simulink model "to_point"  (R2023b)
settings: Solver=FixedStepAuto  StartTime=0.0  StopTime=inf  RelTol=1e-3  EnableMultiTasking=on
model workspace (MAT data in the model file):
  G = 2001
undefined symbols (not defined in the file): c_t, f_max, f_min, Kd, Kp, M, W
libraries: rpi_blkst x2, robotcorelib x1
settings Model: ExtModeTrigDuration=2  Creator=yabde  LastModifiedBy=yabde
settings SolverCC: PositivePriorityOrder=on
settings OptimizationCC: EnhancedBackFolding=on  PassReuseOutputArgsAs=Individual arguments  ZeroExternalMemoryAtStartup=off  ZeroInternalMemoryAtStartup=off  MaxStackSize=64  OptimizeBlockOrder=speed  DifferentSizesBufferReuse=on  OptimizationCustomize=off  EfficientTunableParamExpr=on
settings DebuggingCC: ParameterTunabilityLossMsg=error
settings HardwareCC: ProdBitPerLong=64  ProdLargestAtomicInteger=LongLong  ProdLargestAtomicFloat=Double  ProdLongLongMode=on  ProdHWDeviceType=ARM Compatible->ARM 64-bit (LP64)
settings RTWCC: Description=Embedded Coder  SystemTargetFile=ert.tlc  HardwareBoard=Raspberry Pi (64bit)  TLCOptions="-aInlineSetEventsForThisBaseRateFcn=TLC_FALSE -aSuppressMultiTaskScheduler=TLC_FALSE  -aRateBasedStepFcn=0"  TemplateMakefile=ert_default_tmf  Toolchain=GNU GCC Embedded Linux  BuildConfiguration=Faster Runs
settings CodeAppCC: ForceParamTrailComments=on  IgnoreCustomStorageClasses=off  OperatorAnnotations=on  SimulinkDataObjDesc=on  SFDataObjDesc=on  InsertBlockDesc=on
settings ERTTargetCC: SupportVariableSizeSignals=on  ExtModeTransport=2  ExtModeStaticAlloc=on  ExtModeMexFile=ext_xcp  ExtModeIntrfLevel=Level2 - Open

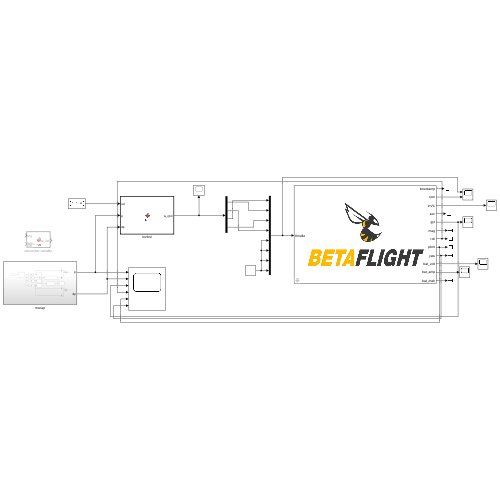
[thumbnail: Simulink's stored preview of the top-level diagram]
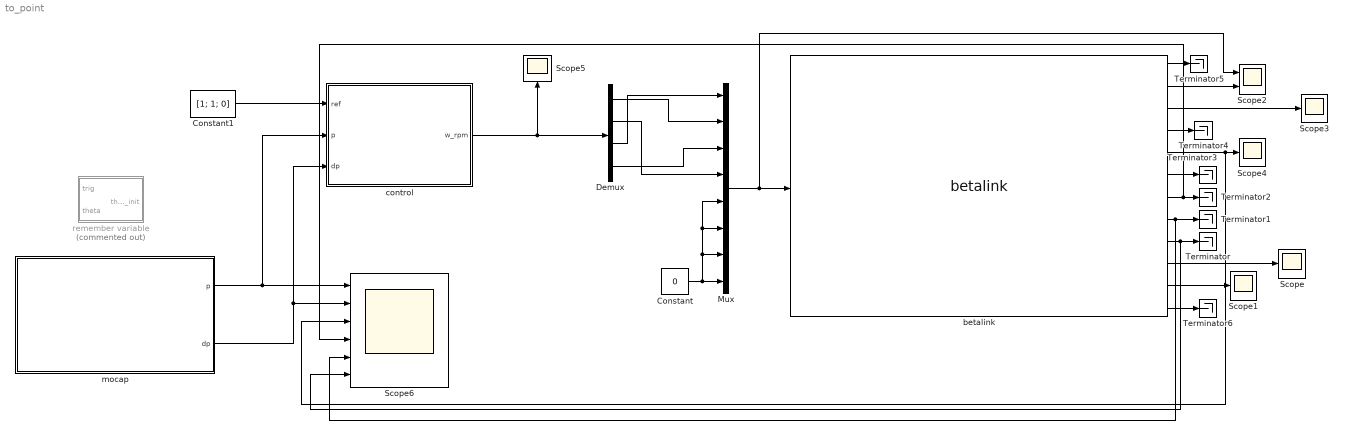
== system to_point ==
  Constant : Constant  Value=0
  Constant1 : Constant  Value=[1; 1; 0]
  Demux : Demux
  Mux : Mux  Inputs=8
  Scope{,1,3..5} (5 alike) : Scope
  Scope2 : Scope  NumInputPorts=2
  Scope6 : Scope  NumInputPorts=6
  Terminator{,1..6} (7 alike) : Terminator
  betalink : rpi_blkst/betalink  rpi_mask_usb_serial_number=1042260556  rpi_mask_Ts=0.01
      settings: SourceProductName=RPI Blockset
  control : MATLAB Function  TreatAsAtomicUnit=on
  mocap : Subsystem
  remember variable : MATLAB Function  Commented=on  TreatAsAtomicUnit=on
  wires:
  Mux/1 -> betalink/1, Scope2/1
  Constant/1 -> Mux/5, Mux/6, Mux/7, Mux/8
  betalink/10 -> Scope/1
  betalink/11 -> Scope1/1
  betalink/2 -> Scope2/2
  betalink/3 -> Scope3/1
  betalink/5 -> Scope6/3, Scope4/1
  betalink/9 -> Scope6/6, Terminator/1
  betalink/8 -> Scope6/5, Terminator1/1
  betalink/7 -> Scope6/4, Terminator2/1
  betalink/6 -> Terminator3/1
  betalink/4 -> Terminator4/1
  betalink/12 -> Terminator6/1
  betalink/1 -> Terminator5/1
  mocap/2(dp) -> control/3(dp), Scope6/2
  control/1(w_rpm) -> Demux/1, Scope5/1
  Demux/1 -> Mux/2
  Demux/2 -> Mux/4
  Demux/3 -> Mux/1
  Demux/4 -> Mux/3
  mocap/1(p) -> control/2(p), Scope6/1
  Constant1/1 -> control/1(ref)

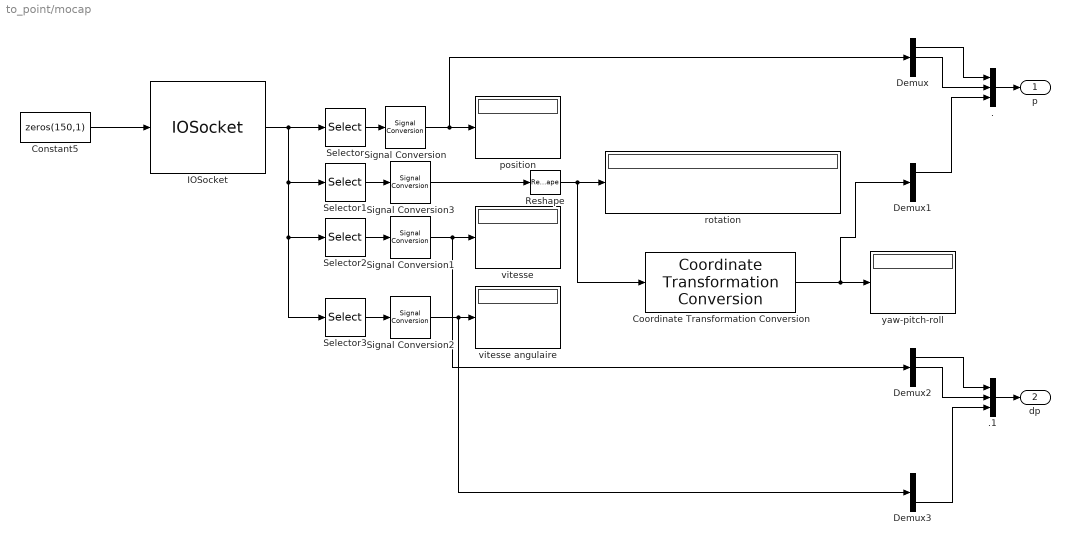
== system to_point/mocap ==
  . : Mux  Inputs=3
  .1 : Mux  Inputs=3
  Constant5 : Constant  Value=zeros(150,1)
  Coordinate Transformation Conversion : robotcorelib/Coordinate Transformation Conversion  InputRepresentation=Rotation Matrix  InputEulerSequence=ZYX  ShowTrVecInputPort=on  OutputRepresentation=Euler Angles  OutputEulerSequence=ZYX  ShowTrVecOutputPort=on  SimulateUsing=Interpreted execution
  Demux{,1..3} (4 alike) : Demux  Outputs=3
  IOSocket : rpi_blkst/IOSocket  rpi_mask_Ts=0.01  rpi_mask_ip1=192  rpi_mask_ip2=168  rpi_mask_ip3=0  rpi_mask_ip4=13  rpi_mask_port=31415
      settings: SourceProductName=RPI Blockset
  Reshape : Reshape  OutputDimensionality=Customize  OutputDimensions=[3,3]
  Selector : Selector  IndexOptions=Index vector (dialog)  Indices=3:5  OutputSizes=1
  Selector1 : Selector  IndexOptions=Index vector (dialog)  Indices=6:14  OutputSizes=1
  Selector2 : Selector  IndexOptions=Index vector (dialog)  Indices=15:17  OutputSizes=1
  Selector3 : Selector  IndexOptions=Index vector (dialog)  Indices=18:20  OutputSizes=1
  Signal Conversion{,1..3} (4 alike) : SignalConversion  OverrideOpt=off
  position : Display
  rotation : Display
  vitesse : Display
  vitesse angulaire : Display
  yaw-pitch-roll : Display
  p : Outport
  dp : Outport  Port=2
  wires:
  Selector2/1 -> Signal Conversion1/1
  Signal Conversion1/1 -> Demux2/1, vitesse/1
  Signal Conversion2/1 -> Demux3/1, vitesse angulaire/1
  Selector/1 -> Signal Conversion/1
  Constant5/1 -> IOSocket/1
  Reshape/1 -> Coordinate Transformation Conversion/1, rotation/1
  IOSocket/1 -> Selector3/1, Selector2/1, Selector1/1, Selector/1
  Selector3/1 -> Signal Conversion2/1
  Signal Conversion/1 -> Demux/1, position/1
  Selector1/1 -> Signal Conversion3/1
  Signal Conversion3/1 -> Reshape/1
  Coordinate Transformation Conversion/1 -> Demux1/1, yaw-pitch-roll/1
  Demux/1 -> ./1
  Demux/2 -> ./2
  Demux1/1 -> ./3
  ./1 -> p/1
  .1/1 -> dp/1
  Demux2/2 -> .1/2
  Demux2/1 -> .1/1
  Demux3/3 -> .1/3

== matlab function to_point/control ==
  data: ref input; w_rpm output size=4; p input; dp input; Kp parameter; Kd parameter; M parameter; W parameter; c_t parameter; f_min parameter; f_max parameter
function w_rpm = fcn(ref,p,dp, Kp, Kd, M, W, c_t, f_min, f_max)

thetaz = wrapToPi(p(3));

Rz = [cos(thetaz), -sin(thetaz), 0; 
      sin(thetaz),  cos(thetaz), 0;
      0,            0,           1];

W_rot = Rz * W;

% Calcul de l'effort souhaité
tau = M * (-Kd * dp + Kp * (ref - p));

% Formulation QP : min ||f||^2 s.t. W_rot*f = tau and fmin <= f <= fmax
H = eye(4);
f_qp = zeros(4,1);

Aeq = W_rot;
beq = tau;

f0 = W_rot \ tau;

% Résolution
options = optimoptions('quadprog', 'Display', 'off', 'Algorithm', 'active-set');
f = quadprog(H, f_qp, [], [], Aeq, beq, f_min, f_max, f0, options);

w = sqrt(f/c_t);

w_rpm = (w * 30/pi); % *1/3 pour avoir des valeurs dans la plage des moteurs

== matlab function to_point/remember variable ==
  data: trig input; theta_init output; theta input
function theta_init = fcn(trig,theta)

persistent theta0 trig_old

if isempty(theta0)
    theta0 = 0;
    trig_old = 0;
end

if trig > trig_old
    theta0 = theta;
end

trig_old = trig;
theta_init = theta0;

end
